simulink model "HW1simulink"  (R2024b)
settings: Solver=FixedStepAuto  StartTime=0.0  StopTime=30  FixedStep=1/86400  RelTol=1e-3
settings Model: Creator=yugpn  LastModifiedBy=JTerr

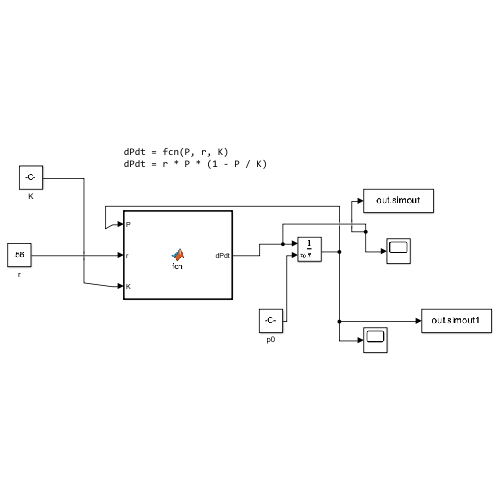
[thumbnail: Simulink's stored preview of the top-level diagram]
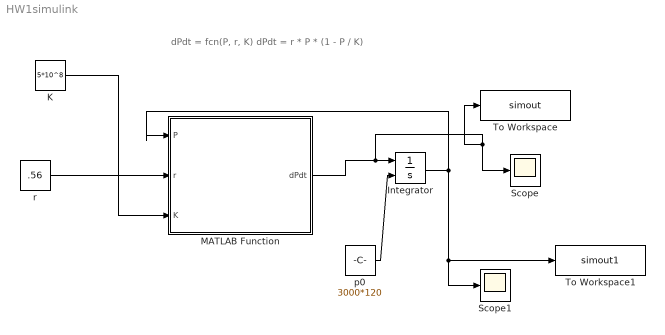
== system HW1simulink ==
  note: dPdt = fcn(P, r, K)
      | dPdt = r * P * (1 - P / K)
  Integrator : Integrator  InitialConditionSource=external
  K : Constant  Value=5*10^8
  MATLAB Function : MATLAB Function  TreatAsAtomicUnit=on
  Scope : Scope
  Scope1 : Scope
  To Workspace : ToWorkspace  VariableName=simout  SampleTime=1
      settings: MaxDataPoints=50  Save2DSignal=2-D array (concatenate along first dimension)
  To Workspace1 : ToWorkspace  VariableName=simout1  SampleTime=1
      settings: MaxDataPoints=50  Save2DSignal=2-D array (concatenate along first dimension)
  p0 : Constant  Value=3000*120
  r : Constant  Value=.56
  wires:
  K/1 -> MATLAB Function/3(K)
  r/1 -> MATLAB Function/2(r)
  p0/1 -> Integrator/2
  Integrator/1 -> MATLAB Function/1(P), To Workspace1/1, Scope1/1
  MATLAB Function/1(dPdt) -> Scope/1, To Workspace/1, Integrator/1

== matlab function HW1simulink/MATLAB Function ==
  data: P input; dPdt output; r input; K input
function dPdt = fcn(P, r, K)
    dPdt = r * P * (1 - P / K);
end
